simulink model "Simulator"  (R2025b)
settings: Solver=FixedStepDiscrete  StartTime=0.0  StopTime=50  FixedStep=0.01  MaxStep=0.1  RelTol=1e-3
values from neighbouring files (symbols this model uses):
  Cd_0 = 0.2    [Interface.m]
  mass = 8    [Interface.m]
  pos0 = [0 0 500]    [Interface.m]
  S_ref = 0.5    [Interface.m]
  v0 = [v0x v0y v0z]    [Interface.m]
  z0 = pos0(3)    [Interface.m]
  z_dir = [0 0 1]    [Interface.m]
undefined symbols (not defined in the file or in its folder): DiscIntNeverNeededParam
settings Model: Creator=mauro  LastModifiedBy=mauro

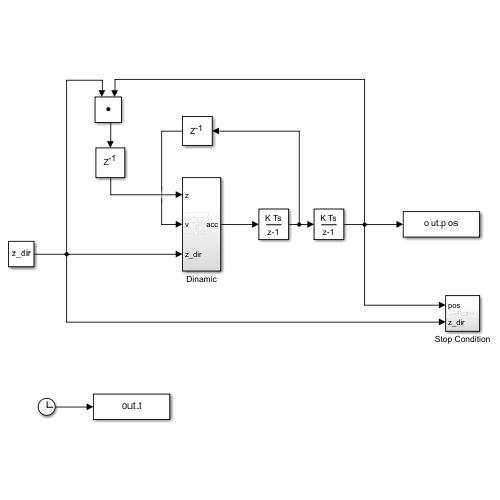
[thumbnail: Simulink's stored preview of the top-level diagram]
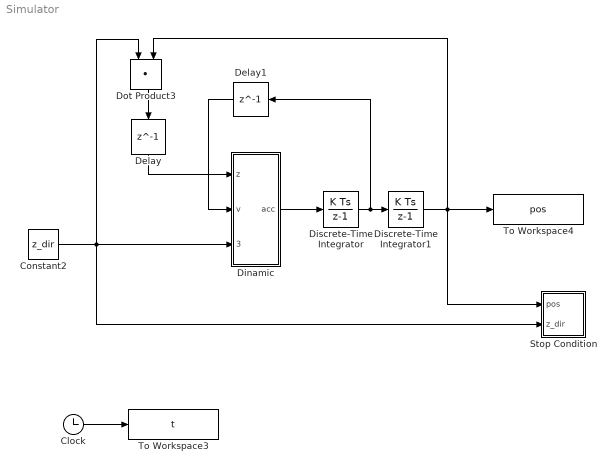
== system Simulator ==
  Clock : Clock
  Constant2 : Constant  Value=z_dir
  Delay : Delay  DelayLength=1  InitialCondition=z0
  Delay1 : Delay  DelayLength=1  InitialCondition=v0
  Dinamic : Subsystem
  Discrete-Time Integrator : DiscreteIntegrator  InitialCondition=v0  SampleTime=-1  ICPrevOutput=DiscIntNeverNeededParam  ICPrevScaledInput=DiscIntNeverNeededParam
  Discrete-Time Integrator1 : DiscreteIntegrator  InitialCondition=pos0  SampleTime=-1  ICPrevOutput=DiscIntNeverNeededParam  ICPrevScaledInput=DiscIntNeverNeededParam
  Dot Product3 : DotProduct  OutDataTypeStr=Inherit: Inherit via internal rule
  Stop Condition : Subsystem
  To Workspace3 : ToWorkspace  VariableName=t  SampleTime=-1
  To Workspace4 : ToWorkspace  VariableName=pos  SampleTime=-1
  wires:
  Clock/1 -> To Workspace3/1
  Constant2/1 -> Dinamic/3(z_dir), Dot Product3/1, Stop Condition/2(z_dir)
  Dinamic/1(acc) -> Discrete-Time Integrator/1
  Discrete-Time Integrator/1 -> Delay1/1, Discrete-Time Integrator1/1
  Discrete-Time Integrator1/1 -> To Workspace4/1, Stop Condition/1(pos), Dot Product3/2
  Dot Product3/1 -> Delay/1
  Delay/1 -> Dinamic/1(z)
  Delay1/1 -> Dinamic/2(v)

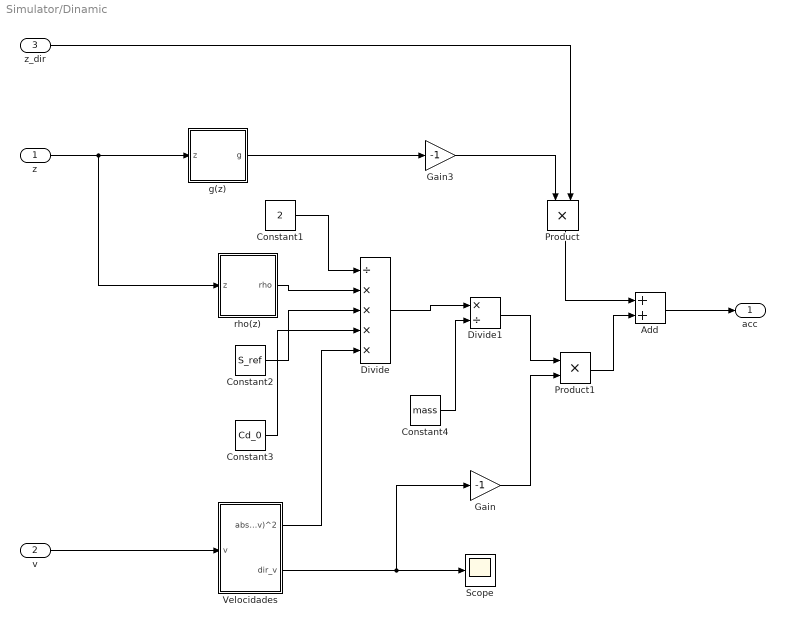
== system Simulator/Dinamic ==
  z : Inport
  v : Inport  Port=2
  z_dir : Inport  Port=3
  Add : Sum
  Constant1 : Constant  Value=2
  Constant2 : Constant  Value=S_ref
  Constant3 : Constant  Value=Cd_0
  Constant4 : Constant  Value=mass
  Divide : Product  Inputs=/****
  Divide1 : Product  Inputs=*/
  Gain : Gain  Gain=-1
  Gain3 : Gain  Gain=-1
  Product : Product
  Product1 : Product
  Scope : Scope
      settings: ActiveDisplayYMinimum=-1.2499870387132885  ActiveDisplayYMaximum=1.2499358103019687
  Velocidades : Subsystem
  g(z) : Subsystem
  rho(z) : Subsystem
  acc : Outport
  wires:
  rho(z)/1(rho) -> Divide/2
  Constant4/1 -> Divide1/2
  Divide/1 -> Divide1/1
  Constant3/1 -> Divide/4
  Constant1/1 -> Divide/1
  Constant2/1 -> Divide/3
  g(z)/1(g) -> Gain3/1
  z/1 -> rho(z)/1(z), g(z)/1(z)
  v/1 -> Velocidades/1(v)
  Velocidades/1(abs(v)^2) -> Divide/5
  Velocidades/2(dir_v) -> Scope/1, Gain/1
  z_dir/1 -> Product/2
  Gain3/1 -> Product/1
  Divide1/1 -> Product1/1
  Gain/1 -> Product1/2
  Product/1 -> Add/1
  Product1/1 -> Add/2
  Add/1 -> acc/1

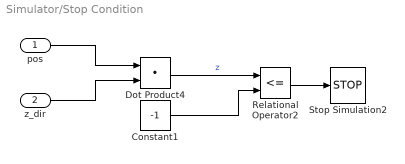
== system Simulator/Stop Condition ==
  pos : Inport
  z_dir : Inport  Port=2
  Constant1 : Constant  Value=-1
  Dot Product4 : DotProduct  OutDataTypeStr=Inherit: Inherit via internal rule
  Relational Operator2 : RelationalOperator  Operator=<=  OutDataTypeStr=boolean  RndMeth=Simplest  InputSameDT=off
  Stop Simulation2 : Stop
  wires:
  pos/1 -> Dot Product4/1
  z_dir/1 -> Dot Product4/2
  Dot Product4/1 -> Relational Operator2/1  "z"
  Relational Operator2/1 -> Stop Simulation2/1
  Constant1/1 -> Relational Operator2/2

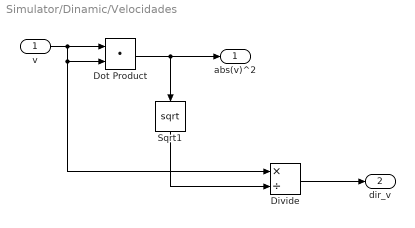
== system Simulator/Dinamic/Velocidades ==
  v : Inport
  Divide : Product  Inputs=*/
  Dot Product : DotProduct  OutDataTypeStr=Inherit: Inherit via internal rule
  Sqrt1 : Sqrt
  abs(v)^2 : Outport
  dir_v : Outport  Port=2
  wires:
  v/1 -> Divide/1, Dot Product/2, Dot Product/1
  Dot Product/1 -> Sqrt1/1, abs(v)^2/1
  Sqrt1/1 -> Divide/2
  Divide/1 -> dir_v/1

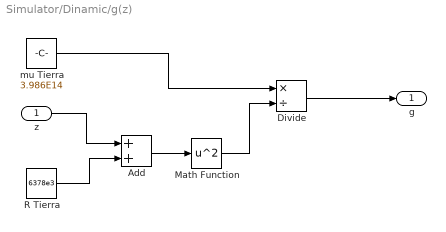
== system Simulator/Dinamic/g(z) ==
  z : Inport
  Add : Sum
  Divide : Product  Inputs=*/
  Math Function : Math  Operator=square
  R Tierra : Constant  Value=6378e3
  mu Tierra : Constant  Value=3.986E14
  g : Outport
  wires:
  Math Function/1 -> Divide/2
  Divide/1 -> g/1
  Add/1 -> Math Function/1
  mu Tierra/1 -> Divide/1
  z/1 -> Add/1
  R Tierra/1 -> Add/2

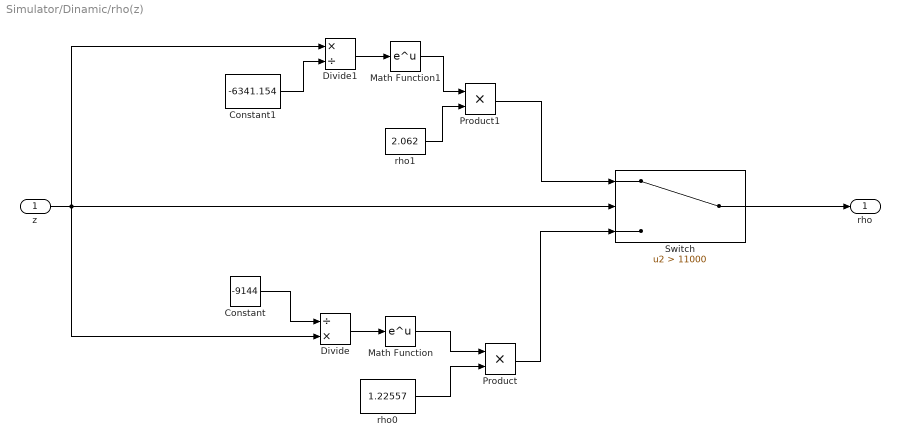
== system Simulator/Dinamic/rho(z) ==
  z : Inport
  Constant : Constant  Value=-9144
  Constant1 : Constant  Value=-6341.154
  Divide : Product  Inputs=/*
  Divide1 : Product  Inputs=*/
  Math Function : Math
  Math Function1 : Math
  Product : Product
  Product1 : Product
  Switch : Switch  Criteria=u2 > Threshold  Threshold=11000  SaturateOnIntegerOverflow=off  InputSameDT=off
  rho0 : Constant  Value=1.22557
  rho1 : Constant  Value=2.062
  rho : Outport
  wires:
  rho0/1 -> Product/2
  Constant/1 -> Divide/1
  Divide/1 -> Math Function/1
  Math Function/1 -> Product/1
  Constant1/1 -> Divide1/2
  z/1 -> Switch/2, Divide1/1, Divide/2
  Divide1/1 -> Math Function1/1
  Math Function1/1 -> Product1/1
  rho1/1 -> Product1/2
  Product1/1 -> Switch/1
  Product/1 -> Switch/3
  Switch/1 -> rho/1
